simulink model "GRP1_Project1_Part2_Model"  (R2013a)
settings: Solver=ode3  StartTime=Time.Start  StopTime=Time.Stop  FixedStep=Time.Step  RelTol=1e-3
values from neighbouring files (symbols this model uses):
  Deq = RH.Deq_temp    [GRP1_Project1_Part2_FINAL.m]
  Height = 200*0.3048    (= 60.96)    [GRP1_Project1_Part2_FINAL.m]
  J = RH.J_temp    [GRP1_Project1_Part2_FINAL.m]
  K = Kmax/2    [GRP1_Project1_Part2_FINAL.m]
  kb = RH.kb_temp    [GRP1_Project1_Part2_FINAL.m]
  kt = RH.kt_temp    [GRP1_Project1_Part2_FINAL.m]
  La = RH.La_temp    [GRP1_Project1_Part2_FINAL.m]
  Ng = RH.Ng_temp    [GRP1_Project1_Part2_FINAL.m]
  Nm = RH.Nm_temp    [GRP1_Project1_Part2_FINAL.m]
  r = RH.r_temp    [GRP1_Project1_Part2_FINAL.m]
  Ra = RH.Ra_temp    [GRP1_Project1_Part2_FINAL.m]
  SimulinkInputSelector = E2.SimulinkInputSelector    [GRP1_Project1_Part2_FINAL.m]
  Tg = E2.Tg    [GRP1_Project1_Part2_FINAL.m]
  UN = 470    [GRP1_Project1_Part2_FINAL.m]
undefined symbols (not defined in the file or in its folder): Time
settings Model: Creator=Nathansen  LastModifiedBy=Nathansen
settings DataIOCC: SaveOutput=off

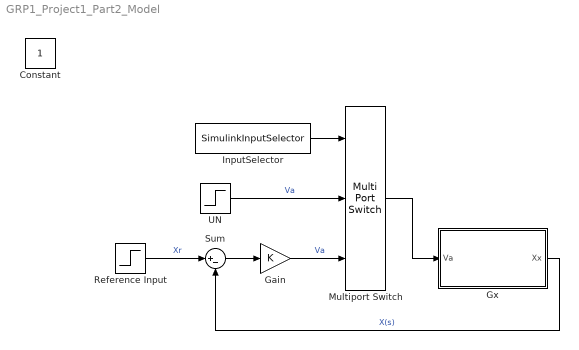
== system GRP1_Project1_Part2_Model ==
  Gain : Gain  Gain=K
  Gx : Subsystem
  InputSelector : Constant  Value=SimulinkInputSelector
  Multiport Switch : MultiPortSwitch  Inputs=2
  Reference Input : Step  Time=0  After=Height  SampleTime=Time.Step
  Sum : Sum  Inputs=|+-
  UN : Step  Time=0  After=UN  SampleTime=Time.Step
  Constant : Constant  IOType=siggen
  wires:
  Gx/1(Xx) -> Sum/2  "X(s)"
  Reference Input/1 -> Sum/1  "Xr"
  Sum/1 -> Gain/1
  Gain/1 -> Multiport Switch/3  "Va"
  Multiport Switch/1 -> Gx/1(Va)
  UN/1 -> Multiport Switch/2  "Va"
  InputSelector/1 -> Multiport Switch/1

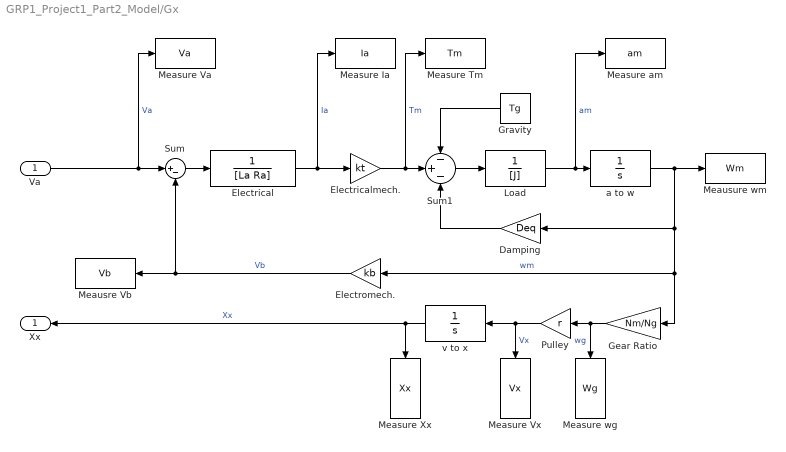
== system GRP1_Project1_Part2_Model/Gx ==
  Va : Inport
  Damping : Gain  Gain=Deq
  Electrical : TransferFcn  Numerator=1  Denominator=[La Ra]
  "Electricalmech. " : Gain  Gain=kt
  Electromech. : Gain  Gain=kb
  Gear Ratio : Gain  Gain=Nm/Ng
  Gravity : Constant  Value=Tg
  Load : TransferFcn  Numerator=1  Denominator=[J]
  Measure Vx : ToWorkspace  VariableName=Vx  SampleTime=-1
  Measure Xx : ToWorkspace  VariableName=Xx  SampleTime=-1
  Measure wg : ToWorkspace  VariableName=Wg  SampleTime=-1
  Measure Ia : ToWorkspace  VariableName=Ia  SampleTime=-1
  Measure Tm : ToWorkspace  VariableName=Tm  SampleTime=-1
  Measure Va : ToWorkspace  VariableName=Va  SampleTime=-1
  Measure am : ToWorkspace  VariableName=am  SampleTime=-1
  Meausre Vb : ToWorkspace  VariableName=Vb  SampleTime=-1
  Meausure wm : ToWorkspace  VariableName=Wm  SampleTime=-1
  Pulley : Gain  Gain=r
  Sum : Sum  Inputs=|+-
  Sum1 : Sum  Inputs=-+-
  a to w : TransferFcn  Numerator=1  Denominator=[1 0]
  v to x : TransferFcn  Numerator=1  Denominator=[1 0]
  Xx : Outport
  wires:
  "Electricalmech. "/1 -> Sum1/2, Measure Tm/1  "Tm"
  Va/1 -> Measure Va/1, Sum/1  "Va"
  Sum1/1 -> Load/1
  Sum/1 -> Electrical/1
  Electrical/1 -> "Electricalmech. "/1, Measure Ia/1  "Ia"
  v to x/1 -> Xx/1, Measure Xx/1  "Xx"
  a to w/1 -> Meausure wm/1, Gear Ratio/1, Electromech./1, Damping/1  "wm"
  Gear Ratio/1 -> Measure wg/1, Pulley/1  "wg"
  Damping/1 -> Sum1/3
  Gravity/1 -> Sum1/1
  Pulley/1 -> v to x/1, Measure Vx/1  "Vx"
  Electromech./1 -> Meausre Vb/1, Sum/2  "Vb"
  Load/1 -> a to w/1, Measure am/1  "am"
